simulink model "SystemARMAX"  (R2023b)
settings: Solver=FixedStepDiscrete  StartTime=0.0  StopTime=tend  RelTol=1e-3  EnableMultiTasking=on
values from neighbouring files (symbols this model uses):
  c1o = 0    [ZAD1.m]
  Td = 1500    [ZAD1.m]
  Tp = 0.1    [ZAD1.m]
libraries: simulink x2
settings Model: Creator=kszygenda  LastModifiedBy=kszygenda
settings SolverCC: AlgebraicLoopSolver=TrustRegion
settings DataIOCC: LimitDataPoints=on  SaveFormat=Array  SignalLoggingSaveFormat=ModelDataLogs  ReturnWorkspaceOutputs=off
settings OptimizationCC: InitFltsAndDblsToZero=on  LifeSpan=inf
settings DebuggingCC: SaveWithParameterizedLinksMsg=none  UnderspecifiedInitializationDetection=Classic  MergeDetectMultiDrivingBlocksExec=none  SignalResolutionControl=TryResolveAllWithWarning  SolverPrmCheckMsg=warning  MultiTaskDSMMsg=warning  MultiTaskCondExecSysMsg=none  FcnCallInpInsideContextMsg=warning  UnconnectedInputMsg=warning  UnconnectedOutputMsg=warning  UnconnectedLineMsg=warning  SFUnexpectedBacktrackingDiag=warning  SFNoUnconditionalDefaultTransitionDiag=warning  SFExecutionAtInitializationDiag=none  ArithmeticOperatorsInVariantConditions=warning
settings HardwareCC: ProdBitPerPointer=32  ProdBitPerSizeT=32  ProdBitPerPtrDiffT=32  ProdLargestAtomicFloat=None  ProdIntDivRoundTo=Undefined  ProdEndianess=Unspecified  ProdWordSize=32  ProdHWDeviceType=32-bit Generic
settings ModelReferenceCC: PropagateSignalLabelsOutOfModel=off
settings CodeAppCC: StateflowObjectComments=on
settings GRTTargetCC: TargetFcnLib=ansi_tfl_tmw.mat  TargetLangStandard=C89/C90 (ANSI)  CombineOutputUpdateFcns=off  GRTInterface=on
settings ConfigComp: CovMetricSettings=dw  CovSaveCumulativeToWorkspaceVar=on  CovSaveSingleToWorkspaceVar=on

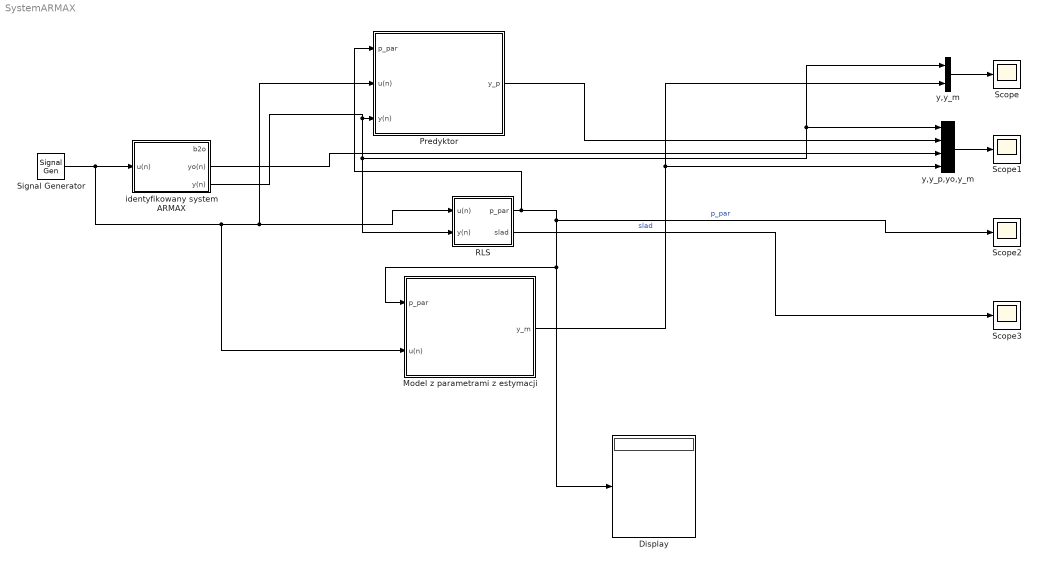
== system SystemARMAX ==
  Display : Display
  Model z parametrami z estymacji : Subsystem
  Predyktor : Subsystem
  RLS : Subsystem
  Scope{,1..3} (4 alike) : Scope
  Signal Generator : SignalGenerator  WaveForm=square  Frequency=0.025
  identyfikowany system ARMAX : Subsystem
  y,y_m : Mux  Inputs=2
  y,y_p,yo,y_m : Mux
  wires:
  Signal Generator/1 -> Model z parametrami z estymacji/2(u(n)), Predyktor/2(u(n)), RLS/1(u(n)), identyfikowany system ARMAX/1(u(n))
  identyfikowany system ARMAX/2(yo(n)) -> y,y_p,yo,y_m/3
  RLS/1(p_par) -> Predyktor/1(p_par), Scope2/1, Display/1, Model z parametrami z estymacji/1(p_par)  "p_par"
  RLS/2(slad) -> Scope3/1  "slad"
  identyfikowany system ARMAX/3(y(n)) -> y,y_p,yo,y_m/1, y,y_m/1, RLS/2(y(n)), Predyktor/3(y(n))
  Model z parametrami z estymacji/1(y_m) -> y,y_p,yo,y_m/4, y,y_m/2
  y,y_m/1 -> Scope/1
  Predyktor/1(y_p) -> y,y_p,yo,y_m/2
  y,y_p,yo,y_m/1 -> Scope1/1

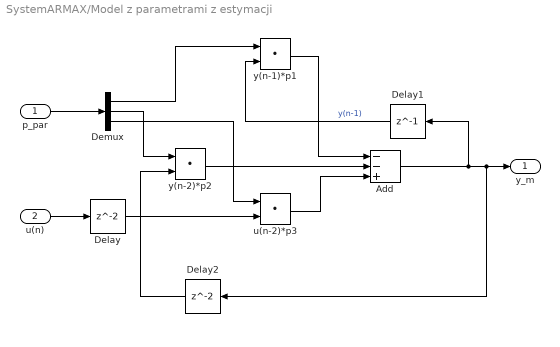
== system SystemARMAX/Model z parametrami z estymacji ==
  p_par : Inport
  u(n) : Inport  Port=2
  Add : Sum  Inputs=--+
  Delay : Delay  InitialCondition=0
  Delay1 : Delay  DelayLength=1  InitialCondition=0
  Delay2 : Delay  InitialCondition=0
  Demux : Demux  Outputs=3
  u(n-2)*p3 : DotProduct  OutDataTypeStr=Inherit: Inherit via internal rule
  y(n-1)*p1 : DotProduct  OutDataTypeStr=Inherit: Inherit via internal rule
  y(n-2)*p2 : DotProduct  OutDataTypeStr=Inherit: Inherit via internal rule
  y_m : Outport
  wires:
  p_par/1 -> Demux/1
  Demux/1 -> y(n-1)*p1/1
  Add/1 -> Delay1/1, Delay2/1, y_m/1
  u(n)/1 -> Delay/1
  Delay/1 -> u(n-2)*p3/2
  Demux/3 -> u(n-2)*p3/1
  u(n-2)*p3/1 -> Add/3
  Delay1/1 -> y(n-1)*p1/2  "y(n-1)"
  y(n-1)*p1/1 -> Add/1
  Demux/2 -> y(n-2)*p2/1
  Delay2/1 -> y(n-2)*p2/2
  y(n-2)*p2/1 -> Add/2

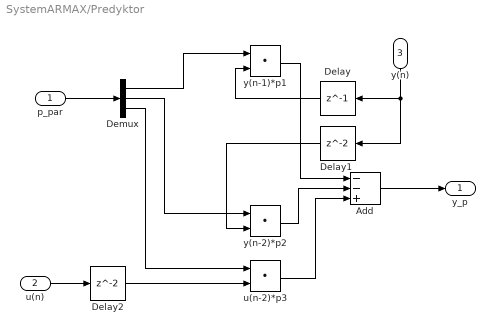
== system SystemARMAX/Predyktor ==
  p_par : Inport
  u(n) : Inport  Port=2
  y(n) : Inport  Port=3
  Add : Sum  Inputs=--+
  Delay : Delay  DelayLength=1  InitialCondition=0
  Delay1 : Delay  InitialCondition=0
  Delay2 : Delay  InitialCondition=0
  Demux : Demux  Outputs=3
  u(n-2)*p3 : DotProduct  OutDataTypeStr=Inherit: Inherit via internal rule
  y(n-1)*p1 : DotProduct  OutDataTypeStr=Inherit: Inherit via internal rule
  y(n-2)*p2 : DotProduct  OutDataTypeStr=Inherit: Inherit via internal rule
  y_p : Outport
  wires:
  p_par/1 -> Demux/1
  Demux/1 -> y(n-1)*p1/1
  Demux/2 -> y(n-2)*p2/1
  Demux/3 -> u(n-2)*p3/1
  Delay/1 -> y(n-1)*p1/2
  Delay1/1 -> y(n-2)*p2/2
  u(n)/1 -> Delay2/1
  Delay2/1 -> u(n-2)*p3/2
  y(n-1)*p1/1 -> Add/1
  u(n-2)*p3/1 -> Add/3
  y(n-2)*p2/1 -> Add/2
  Add/1 -> y_p/1
  y(n)/1 -> Delay/1, Delay1/1

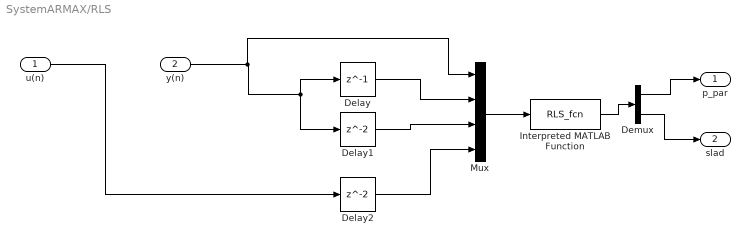
== system SystemARMAX/RLS ==
  u(n) : Inport
  y(n) : Inport  Port=2
  Delay : Delay  DelayLength=1  InitialCondition=0
  Delay1 : Delay  InitialCondition=0
  Delay2 : Delay  InitialCondition=0
  Demux : Demux  Outputs=[3;1]
  Interpreted MATLAB Function : MATLABFcn  MATLABFcn=RLS_fcn  OutputDimensions=4
  Mux : Mux
  p_par : Outport
  slad : Outport  Port=2
  wires:
  u(n)/1 -> Delay2/1
  y(n)/1 -> Mux/1, Delay1/1, Delay/1
  Delay/1 -> Mux/2
  Demux/2 -> slad/1
  Delay1/1 -> Mux/3
  Delay2/1 -> Mux/4
  Interpreted MATLAB Function/1 -> Demux/1
  Demux/1 -> p_par/1
  Mux/1 -> Interpreted MATLAB Function/1

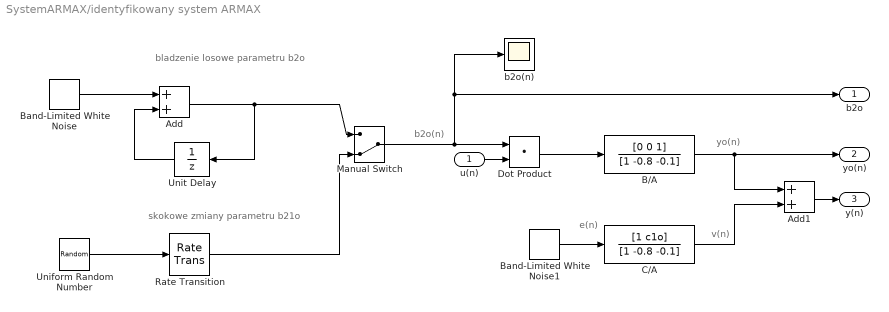
== system SystemARMAX/identyfikowany system ARMAX ==
  note: e(n)
  note: v(n)
  note: yo(n)
  note: b2o(n)
  note: skokowe zmiany parametru b21o
  note: bladzenie losowe parametru b2o
  u(n) : Inport
  Add : Sum
  Add1 : Sum
  B/A : DiscreteFilter  Numerator=[0 0 1]  Denominator=[1 -0.8 -0.1]  SampleTime=Tp
  Band-Limited White Noise : simulink/Sources/Band-Limited White Noise  Cov=[0.00001*Tp]  Ts=Tp  seed=[23341]
  Band-Limited White Noise1 : simulink/Sources/Band-Limited White Noise  Cov=[0.001*Tp]  Ts=Tp  seed=[23341]
  C/A : DiscreteFilter  Numerator=[1 c1o]  Denominator=[1 -0.8 -0.1]  SampleTime=Tp
  Dot Product : DotProduct  OutDataTypeStr=Inherit: Inherit via internal rule
  Manual Switch : ManualSwitch  CurrentSetting=0
  Rate Transition : RateTransition  InitialCondition=0.5  OutPortSampleTime=Tp
  Uniform Random Number : UniformRandomNumber  Minimum=0.1  Maximum=0.8  Seed=2  SampleTime=Td
  Unit Delay : UnitDelay  SampleTime=Tp
  b2o(n) : Scope
  b2o : Outport
  yo(n) : Outport  Port=2
  y(n) : Outport  Port=3
  wires:
  Band-Limited White Noise/1 -> Add/1
  Add/1 -> Unit Delay/1, Manual Switch/1
  Unit Delay/1 -> Add/2
  Uniform Random Number/1 -> Rate Transition/1
  Rate Transition/1 -> Manual Switch/2
  Manual Switch/1 -> Dot Product/1, b2o/1, b2o(n)/1
  Dot Product/1 -> B/A/1
  C/A/1 -> Add1/2
  B/A/1 -> Add1/1, yo(n)/1
  Band-Limited White Noise1/1 -> C/A/1
  u(n)/1 -> Dot Product/2
  Add1/1 -> y(n)/1
